simulink model "T3_A_sim"  (R2024b)
settings: Solver=VariableStepAuto  StartTime=0.0  StopTime=10.0  RelTol=1e-3

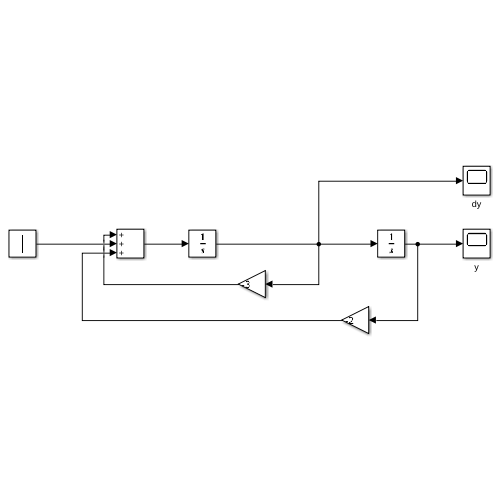
[thumbnail: Simulink's stored preview of the top-level diagram]
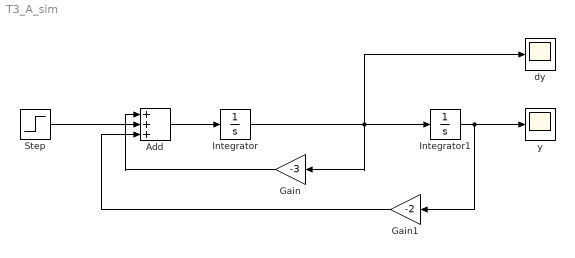
== system T3_A_sim ==
  Add : Sum  Inputs=+++
  Gain : Gain  Gain=-3
  Gain1 : Gain  Gain=-2
  Integrator : Integrator
  Integrator1 : Integrator
  Step : Step  Time=0  SampleTime=0
  dy : Scope
  y : Scope
  wires:
  Step/1 -> Add/2
  Add/1 -> Integrator/1
  Integrator/1 -> dy/1, Gain/1, Integrator1/1
  Integrator1/1 -> Gain1/1, y/1
  Gain/1 -> Add/1
  Gain1/1 -> Add/3
